simulink model "Conventional_Buck_GateSignal_SWdebounce"  (R2017b)
settings: Solver=ode1  StartTime=0.0  StopTime=2e-3  FixedStep=Ts  RelTol=1e-3
PostLoadFcn:
  | , if any(exist('dsrtsu_mdlpostloadfcn', 'file') == [2, 3, 6]), try dsrtsu_mdlpostloadfcn('Execute', bdroot); catch fprintf('Error in PostLoadFcn (dsrtsu_mdlpostloadfcn) for model "%s":\n %s\n', bdroot, lasterr); end, end,
values from neighbouring files (symbols this model uses):
  Ts = 10e-9    (= 1e-08)    [init_conventional_buck.m]
  Vin = 12    [init_conventional_buck.m]
  Vmax = 10    [init_conventional_buck.m]
  Vref = 3.3    [init_conventional_buck.m]
libraries: simulink x3
Description:
  | Standard RTI1005 template.
  | Supported MATLAB version:  R2017b.
settings Model: Tag=RTI1005  DSRTSU_INTERNAL_RTI_VER=540  DSRTSU_INTERNAL_RTI_TYPE=rti1005  RTICANMMDATA=struct('GeneralSetupData',struct('modelroot','C:\Projects\Simulink\PE_1\w3','generalsettings',struct('filesettings',struct('destfolder',struct('Name','RTICANMM_FILES','Check',1),'buildfolder',struct('Name','.','Check',1),'AbsDestfolder',struct('Name','C:\Projects\Simulink\PE_1\w3\RTICANMM_FILES'),'AbsBuildfolder',struct('Name','C:\Projects\Simulink\PE_1\w3'))),'options',struct('addpaths',1,'rmpaths',1,'addtrcexclusion',logical(1),'cannavigator',struct('checkmonitoring',0),'show_usrtrc',0,'use_usrtrc',0),'advanced',struct('options',ones(1,100)),'MPSetup',{{}},'RTI',struct('Type','RTI1005','Ver','7.12','Date','02-May-2019'),'modelname','conv_buck_dutyCalc_switch_debounce','block','conv_buck_dutyCalc_switch_debounce'))  DSRTSU_INTERNAL_RTIFPGA=130  Creator=CA72672  LastModifiedBy=CA72672
settings OptimizationCC: BlockReduction=off  OptimizeBlockIOStorage=off  BufferReuse=off  GlobalBufferReuse=off  ExpressionFolding=off  LocalBlockOutputs=off
settings HardwareCC: ProdBitPerPointer=32  ProdBitPerSizeT=32  ProdBitPerPtrDiffT=32  ProdLargestAtomicInteger=Integer  ProdEndianess=BigEndian  ProdWordSize=32  ProdHWDeviceType=Custom Processor->Custom  TargetIntDivRoundTo=Zero  TargetEndianess=BigEndian  TargetHWDeviceType=Custom Processor->Custom
settings SFSimCC: MATLABDynamicMemAlloc=off
settings RTWCC: SystemTargetFile=rti1005.tlc  MakeCommand=make_rti  TemplateMakefile=rti1005.tmf  Description=dSPACE DS1005 Hardware Platform
settings CodeAppCC: StateflowObjectComments=on
settings STFCustomTargetCC: ParMdlRefBuildCompliant=on  MatFileLogging=on  GRTInterface=off  SystemTargetFile=rti1005.tlc
settings GRTTargetCC: TargetLangStandard=C89/C90 (ANSI)  CompOptLevelCompliant=off  ConcurrentExecutionCompliant=off  CombineOutputUpdateFcns=off  CPPClassGenCompliant=off  UseToolchainInfoCompliant=off
settings ConfigComp: CovMetricSettings=dswe

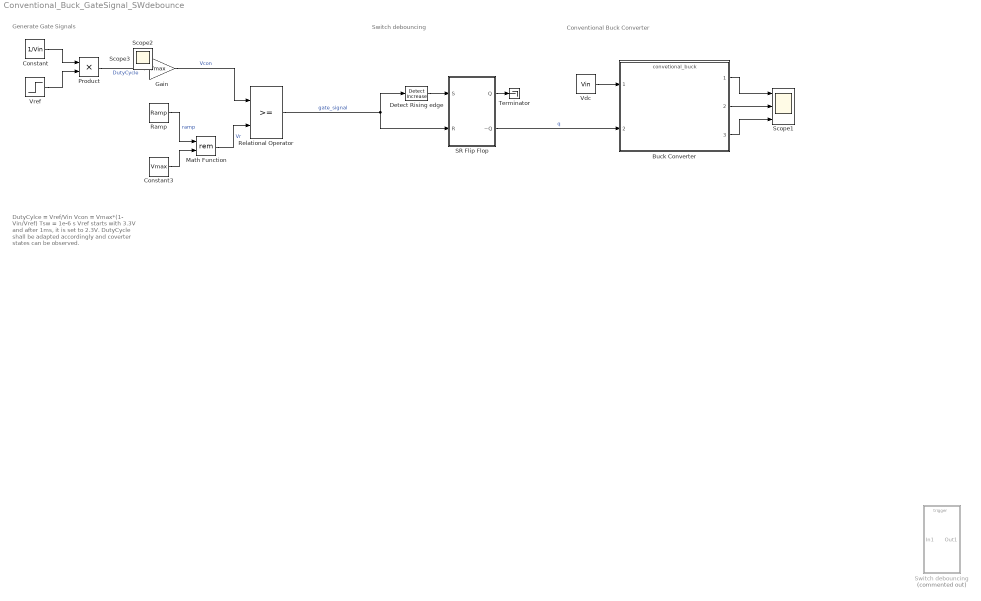
== system Conventional_Buck_GateSignal_SWdebounce ==
  note: DutyCylce = Vref/Vin
      |
      | Vcon = Vmax*(1- Vin/Vref)
      |
      | Tsw = 1e-6 s
      |
      | Vref starts with 3.3V and after 1ms, it is set to 2.3V.
      | DutyCycle shall be adapted accordingly and coverter states can be observed.
  note: Conventional Buck Converter
  note: Switch debouncing
  note: Generate Gate Signals
  Buck Converter : ModelReference  ModelNameDialog=convetional_buck.slx  SimulationMode=Normal  ModelReferenceVersion=1.31
  Constant : Constant  Value=1/Vin
  Constant3 : Constant  Value=Vmax
  Detect Rising edge : simulink/Logic and Bit Operations/Detect Increase  vinit=0.0  OutDataTypeStr=boolean
  Gain : Gain  Gain=Vmax
  Math Function : Math  Operator=rem  SaturateOnIntegerOverflow=on
  Product : Product
  Ramp : simulink/Sources/Ramp  slope=Vmax/Tsw  start=0  X0=0
  Relational Operator : RelationalOperator  OutDataTypeStr=boolean  RndMeth=Simplest
  SR Flip Flop : Subsystem
  Scope1 : Scope  NumInputPorts=3
  Switch debouncing : Subsystem  Commented=on  TreatAsAtomicUnit=on
  Terminator : Terminator
  Vdc : Constant  Value=Vin
  Vref : Step  Time=1.05e-3  Before=Vref  After=Vref-1
  Scope2 : Scope
  Scope3 : Scope
  wires:
  Vref/1 -> Product/2
  Constant/1 -> Product/1
  Product/1 -> Gain/1  "DutyCycle"
  Gain/1 -> Relational Operator/1  "Vcon"
  Ramp/1 -> Math Function/1  "ramp"
  Constant3/1 -> Math Function/2
  Math Function/1 -> Relational Operator/2  "Vr"
  Relational Operator/1 -> Detect Rising edge/1, SR Flip Flop/2(R)  "gate_signal"
  Vdc/1 -> Buck Converter/1
  Detect Rising edge/1 -> SR Flip Flop/1(S)
  Buck Converter/2 -> Scope1/2
  Buck Converter/1 -> Scope1/1
  Buck Converter/3 -> Scope1/3
  SR Flip Flop/2(~Q) -> Buck Converter/2  "q"
  SR Flip Flop/1(Q) -> Terminator/1

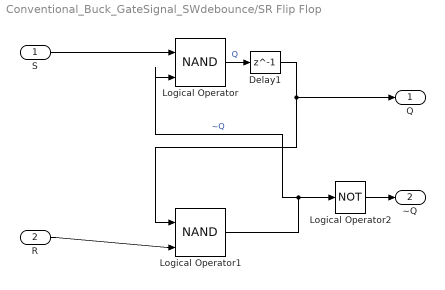
== system Conventional_Buck_GateSignal_SWdebounce/SR Flip Flop ==
  S : Inport
  R : Inport  Port=2
  Delay1 : Delay  DelayLength=1
  Logical Operator : Logic  Operator=NAND  IconShape=distinctive  AllPortsSameDT=off  OutDataTypeStr=boolean
  Logical Operator1 : Logic  Operator=NAND  IconShape=distinctive  AllPortsSameDT=off  OutDataTypeStr=boolean
  Logical Operator2 : Logic  Operator=NOT  IconShape=distinctive  AllPortsSameDT=off  OutDataTypeStr=boolean
  Q : Outport
  ~Q : Outport  Port=2
  wires:
  Delay1/1 -> Q/1, Logical Operator1/1
  S/1 -> Logical Operator/1
  R/1 -> Logical Operator1/2
  Logical Operator/1 -> Delay1/1  "Q"
  Logical Operator1/1 -> Logical Operator2/1, Logical Operator/2  "~Q"
  Logical Operator2/1 -> ~Q/1

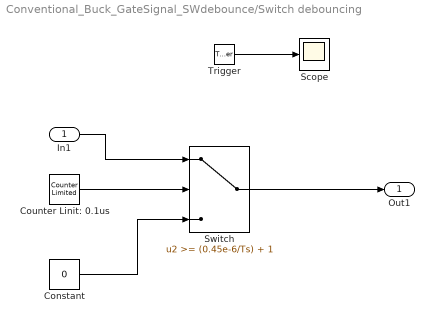
== system Conventional_Buck_GateSignal_SWdebounce/Switch debouncing ==
  In1 : Inport
  Trigger : TriggerPort  VariantControl=Variant  ShowOutputPort=on  PortDimensions=1
  Constant : Constant  Value=0
  Counter Linit: 0.1us : simulink/Sources/Counter Limited  uplimit=(0.45e-6/Ts) + 1  tsamp=-1
  Scope : Scope
  Switch : Switch  Threshold=(0.45e-6/Ts) + 1
  Out1 : Outport
  wires:
  In1/1 -> Switch/1
  Switch/1 -> Out1/1
  Counter Linit: 0.1us/1 -> Switch/2
  Constant/1 -> Switch/3
  Trigger/1 -> Scope/1
